simulink model "W07_0_offline"  (R2024b)
settings: Solver=ode4  StartTime=0.0  StopTime=600  FixedStep=Ts_ctrl  RelTol=1e-3
values from neighbouring files (symbols this model uses):
  animate = 0    [W05_compare.m]    (also in W05_crab_demo.m; W05_lookahead_demo.m; W05_setup.m = 1; W07_setup.m = 1)
  beta_c = deg2rad(current_direction)    [W05_compare.m]    (also in W05_crab_demo.m; W05_setup.m; W07_setup.m)
  current_speed = CASES{i,3}    [W05_compare.m]    (also in W05_crab_demo.m = CUR(i); W05_setup.m = 0; W07_setup.m = 0)
  d_mode = 1    [W07_setup.m]
  Delta = DELTAS(i)    [W05_lookahead_demo.m]    (also in W05_setup.m = 10; W07_setup.m = 10)
  F_max = 500    [W05_setup.m]    (also in W07_setup.m)
  guidance_mode = CASES{i,2}    [W05_compare.m]    (also in W05_setup.m = 2; W07_setup.m = 2)
  half_beam = 1.027135    [W05_setup.m]    (also in W07_setup.m)
  Izz = 653    [W05_setup.m]    (also in W07_setup.m; build_w05_models.m = p(2))
  k_prop = 1000 * 0.004422 * 0.2^4    (= 0.0070752)    [W05_setup.m]    (also in W07_setup.m)
  Kd_psi = 200    [W05_setup.m]    (also in W07_setup.m)
  Ki_u = 100    [W05_setup.m]    (also in W07_setup.m)
  Kp_psi = 400    [W05_setup.m]    (also in W07_setup.m)
  Kp_u = 300    [W05_setup.m]    (also in W07_setup.m)
  m_usv = 211    [W05_setup.m]    (also in W07_setup.m)
  n_max = sqrt(F_max / k_prop)    [W05_setup.m]    (also in W07_setup.m)
  Nr = 800    [W05_setup.m]    (also in W07_setup.m)
  Nrr = 800    [W05_setup.m]    (also in W07_setup.m; build_w05_models.m = p(8))
  R_LOS = 5    [W05_lookahead_demo.m]    (also in W05_setup.m; W07_setup.m)
  sw_mode = 1    [W05_lookahead_demo.m]    (also in W05_setup.m; W07_setup.m)
  tau_n = 0.30    (= 0.3)    [W05_setup.m]    (also in W07_setup.m)
  Ts_ctrl = 0.05    [W05_setup.m]    (also in W07_setup.m)
  u_ref = 1.5    [W05_setup.m]    (also in W07_setup.m)
  wp_east = [  20   20  100  100   20 ]    [W05_setup.m]    (also in W07_setup.m)
  wp_north = [ -20   60   60  -20  -20 ]    [W05_setup.m]    (also in W07_setup.m)
  x0 = [0.1; 0; 0; 0; 0; psi_init]    [W05_setup.m]    (also in W05_vrx_run.m = x0old;   x0(6) = psi0;   assignin('base','x0', x0); W07_setup.m)
  Xu = 100    [W05_setup.m]    (also in W07_setup.m; build_w05_models.m = p(3))
  Xuu = 150    [W05_setup.m]    (also in W07_setup.m; build_w05_models.m = p(4))
  Yv = 100    [W05_setup.m]    (also in W07_setup.m; build_w05_models.m = p(5))
  Yvv = 100    [W05_setup.m]    (also in W07_setup.m; build_w05_models.m = p(6);'                newline  'Nr=p(7))
libraries: slpidlib x1, simulink x1
settings Model: Creator=admin  LastModifiedBy=admin

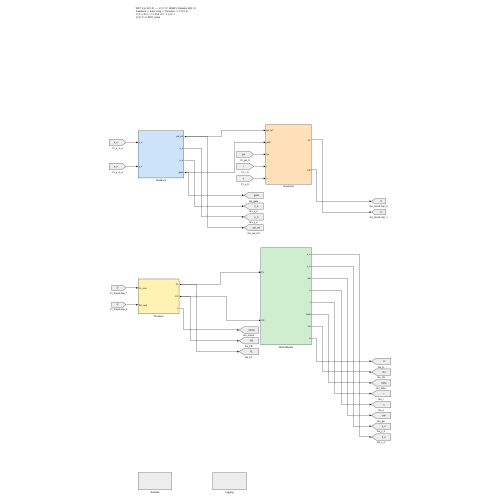
[thumbnail: Simulink's stored preview of the top-level diagram]
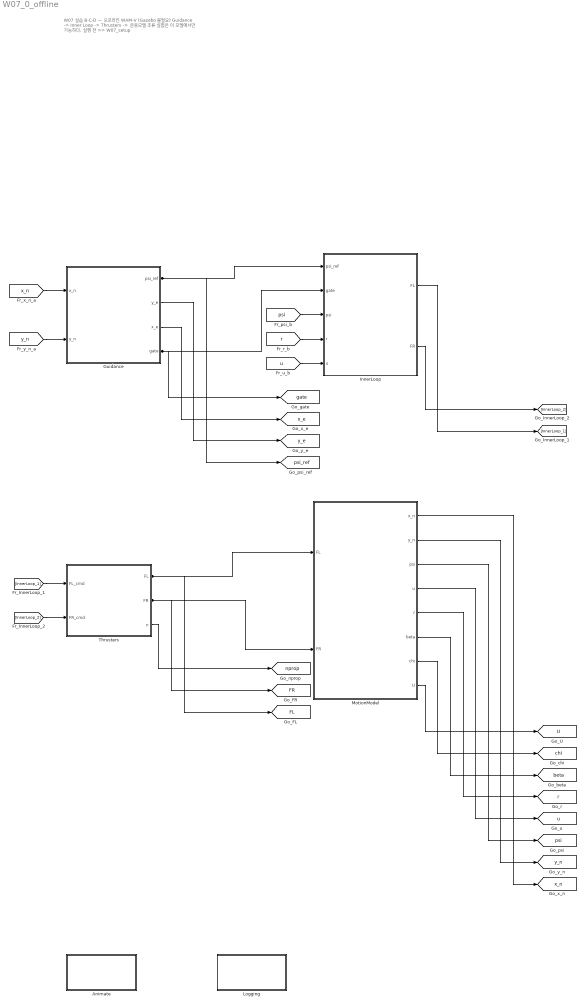
== system W07_0_offline ==
  note: W07 실습 B·C·D  —  오프라인 WAM-V (Gazebo 불필요)
      | Guidance -> Inner Loop -> Thrusters -> 운동모델
      | 조류 실험은 이 모델에서만 가능하다.
      | 실행 전 >> W07_setup
  Animate : Subsystem
  Guidance : Subsystem
  InnerLoop : Subsystem
  Logging : Subsystem
  MotionModel : Subsystem
  Thrusters : Subsystem
  tag scope: FL=global, FR=global, U=global, beta=global, chi=global, gate=global, nprop=global, psi=global, psi_ref=global, r=global, u=global, x_e=global, x_n=global, y_e=global, y_n=global
  wires:
  MotionModel/8(U) -> [U]
  MotionModel/7(chi) -> [chi]
  MotionModel/6(beta) -> [beta]
  MotionModel/5(r) -> [r]
  MotionModel/4(u) -> [u]
  MotionModel/3(psi) -> [psi]
  MotionModel/2(y_n) -> [y_n]
  MotionModel/1(x_n) -> [x_n]
  InnerLoop/2(FR) -> [InnerLoop_2]
  InnerLoop/1(FL) -> [InnerLoop_1]
  Thrusters/3(n) -> [nprop]
  Thrusters/2(FR) -> MotionModel/2(FR), [FR]
  Thrusters/1(FL) -> MotionModel/1(FL), [FL]
  [u] -> InnerLoop/5(u)
  [r] -> InnerLoop/4(r)
  [psi] -> InnerLoop/3(psi)
  Guidance/4(gate) -> InnerLoop/2(gate), [gate]
  Guidance/3(x_e) -> [x_e]
  Guidance/2(y_e) -> [y_e]
  Guidance/1(psi_ref) -> InnerLoop/1(psi_ref), [psi_ref]
  [y_n] -> Guidance/2(y_n)
  [x_n] -> Guidance/1(x_n)
  [InnerLoop_2] -> Thrusters/2(FR_cmd)
  [InnerLoop_1] -> Thrusters/1(FL_cmd)

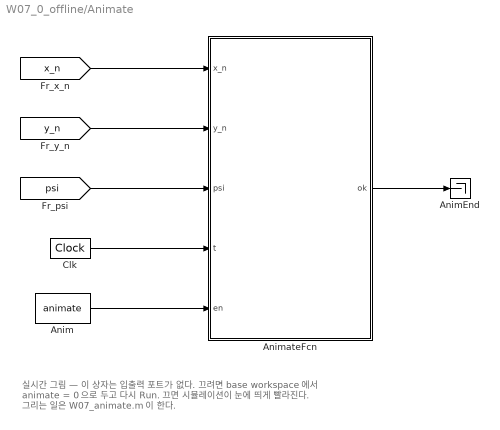
== system W07_0_offline/Animate ==
  note: 실시간 그림 — 이 상자는 입출력 포트가 없다.
      | 끄려면 base workspace 에서  animate = 0  으로 두고 다시 Run.
      | 끄면 시뮬레이션이 눈에 띄게 빨라진다.
      | 그리는 일은 W07_animate.m 이 한다.
  Anim : Constant  Value=animate
  AnimEnd : Terminator
  AnimateFcn : MATLAB Function  TreatAsAtomicUnit=on
  Clk : DigitalClock  SampleTime=Ts_ctrl
  wires:
  [x_n] -> AnimateFcn/1(x_n)
  [y_n] -> AnimateFcn/2(y_n)
  [psi] -> AnimateFcn/3(psi)
  Clk/1 -> AnimateFcn/4(t)
  Anim/1 -> AnimateFcn/5(en)
  AnimateFcn/1(ok) -> AnimEnd/1

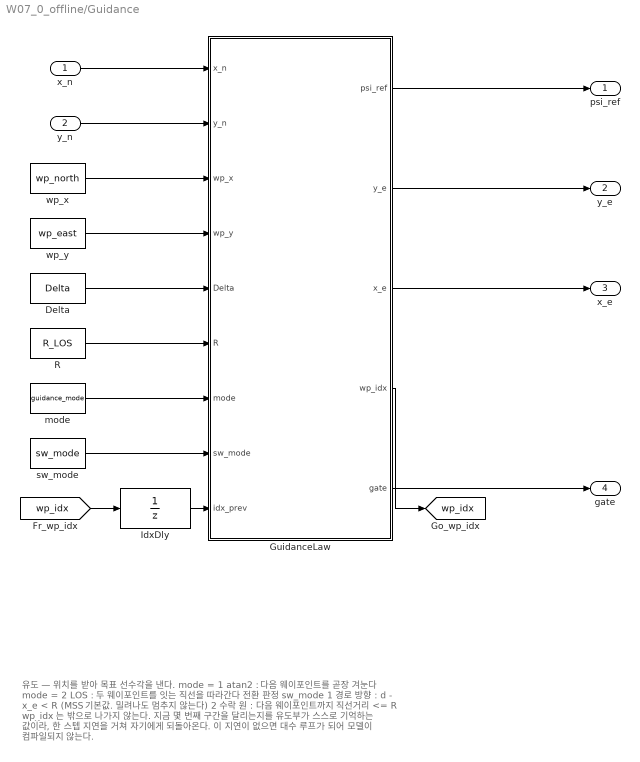
== system W07_0_offline/Guidance ==
  note: 유도 — 위치를 받아 목표 선수각을 낸다.
      |   mode = 1  atan2 : 다음 웨이포인트를 곧장 겨눈다
      |   mode = 2  LOS   : 두 웨이포인트를 잇는 직선을 따라간다
      |
      | 전환 판정 sw_mode
      |   1  경로 방향 : d - x_e < R   (MSS 기본값. 밀려나도 멈추지 않는다)
      |   2  수락 원   : 다음 웨이포인트까지 직선거리 <= R
      |
      | wp_idx 는 밖으로 나가지 않는다. 지금 몇 번째 구간을 달리는지를
      | 유도부가 스스로 기억하는 값이라, 한 스텝 지연을 거쳐 자기에게 되돌아온다.
      | 이 지연이 없으면 대수 루프가 되어 모델이 컴파일되지 않는다.
  x_n : Inport
  y_n : Inport  Port=2
  Delta : Constant  Value=Delta
  GuidanceLaw : MATLAB Function  TreatAsAtomicUnit=on
  IdxDly : UnitDelay  InitialCondition=1  SampleTime=Ts_ctrl  HasFrameUpgradeWarning=on
  R : Constant  Value=R_LOS
  mode : Constant  Value=guidance_mode
  sw_mode : Constant  Value=sw_mode
  wp_x : Constant  Value=wp_north
  wp_y : Constant  Value=wp_east
  psi_ref : Outport
  y_e : Outport  Port=2
  x_e : Outport  Port=3
  gate : Outport  Port=4
  tag scope: wp_idx=global
  wires:
  x_n/1 -> GuidanceLaw/1(x_n)
  y_n/1 -> GuidanceLaw/2(y_n)
  wp_x/1 -> GuidanceLaw/3(wp_x)
  wp_y/1 -> GuidanceLaw/4(wp_y)
  Delta/1 -> GuidanceLaw/5(Delta)
  R/1 -> GuidanceLaw/6(R)
  mode/1 -> GuidanceLaw/7(mode)
  sw_mode/1 -> GuidanceLaw/8(sw_mode)
  [wp_idx] -> IdxDly/1
  IdxDly/1 -> GuidanceLaw/9(idx_prev)
  GuidanceLaw/1(psi_ref) -> psi_ref/1
  GuidanceLaw/2(y_e) -> y_e/1
  GuidanceLaw/3(x_e) -> x_e/1
  GuidanceLaw/5(gate) -> gate/1
  GuidanceLaw/4(wp_idx) -> [wp_idx]

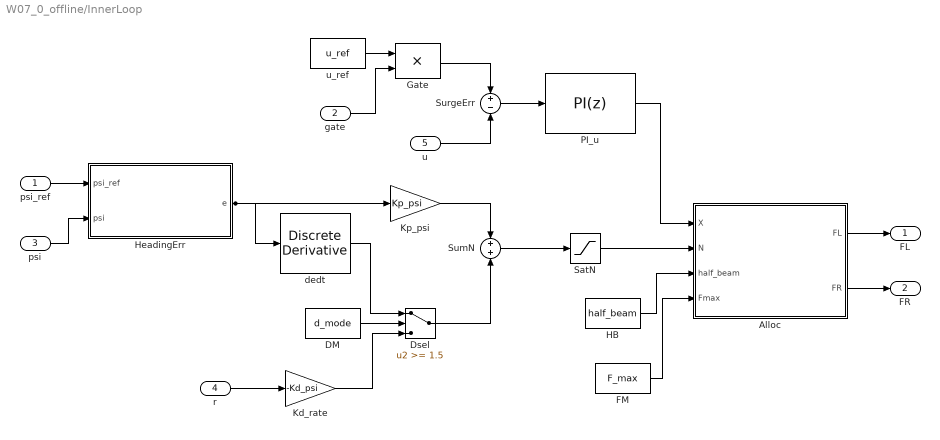
== system W07_0_offline/InnerLoop ==
  psi_ref : Inport
  gate : Inport  Port=2
  psi : Inport  Port=3
  r : Inport  Port=4
  u : Inport  Port=5
  Alloc : MATLAB Function  TreatAsAtomicUnit=on
  DM : Constant  Value=d_mode
  Dsel : Switch  Threshold=1.5  SaturateOnIntegerOverflow=off  InputSameDT=off
  FM : Constant  Value=F_max
  Gate : Product
  HB : Constant  Value=half_beam
  HeadingErr : MATLAB Function  TreatAsAtomicUnit=on
  Kd_rate : Gain  Gain=-Kd_psi
  Kp_psi : Gain  Gain=Kp_psi
  PI_u : slpidlib/PID Controller  Controller=PI  Form=Parallel  TimeDomain=Discrete-time  UseExternalTs=off  SampleTime=Ts_ctrl  IntegratorMethod=Forward Euler  FilterMethod=Forward Euler  ControllerParametersSource=internal  P=Kp_u  I=Ki_u  UseKiTs=off  D=0  UseExternalDerivativeSource=off  N=100  UseFilter=on  TunerSelectOption=Transfer Function Based (PID Tuner App)  InitialConditionSource=internal  InitialConditionForIntegrator=0  InitialConditionForFilter=0  DifferentiatorICPrevScaledInput=0  ExternalReset=none  TrackingMode=off  Kt=1  LimitOutput=on  SatLimitsSource=internal  UpperSaturationLimit=2*F_max  LowerSaturationLimit=-2*F_max  LinearizeAsGain=on  AntiWindupMode=clamping  Kb=1  LimitIntegrator=off  UpperIntegratorSaturationLimit=inf  LowerIntegratorSaturationLimit=-inf  POutMin=[]  POutMax=[]  IOutMin=[]  IOutMax=[]  DOutMin=[]  DOutMax=[]  NOutMin=[]  NOutMax=[]  SumOutMin=[]  SumOutMax=[]  SaturationOutMin=[]  SaturationOutMax=[]  PParamMin=[]  PParamMax=[]  IParamMin=[]  IParamMax=[]  DParamMin=[]  DParamMax=[]  NParamMin=[]  NParamMax=[]  KbParamMin=[]  KbParamMax=[]  KtParamMin=[]  KtParamMax=[]  KbOutMin=[]  KbOutMax=[]  KtOutMin=[]  KtOutMax=[]  IntegratorOutMin=[]  IntegratorOutMax=[]  FilterOutMin=[]  FilterOutMax=[]  SumI1OutMin=[]  SumI1OutMax=[]  SumI2OutMin=[]  SumI2OutMax=[]  SumI3OutMin=[]  SumI3OutMax=[]  SumI4OutMin=[]  SumI4OutMax=[]  SumDOutMin=[]  SumDOutMax=[]  DifferentiatorOutMin=[]  DifferentiatorOutMax=[]  FilterDiffOutCoefMin=[]  FilterDiffOutCoefMax=[]  ReciprocalOutMin=[]  ReciprocalOutMax=[]  SumDenOutMin=[]  SumDenOutMax=[]  SumNumOutMin=[]  SumNumOutMax=[]  DivideOutMin=[]  DivideOutMax=[]  UdiffTsProdOutMin=[]  UdiffTsProdOutMax=[]  NTsProdOutMin=[]  NTsProdOutMax=[]  UintegralTsProdOutMin=[]  UintegralTsProdOutMax=[]  UngainTsProdOutMin=[]  UngainTsProdOutMax=[]  ClampingZeroOutDataTypeStr=Inherit: Inherit via back propagation  ClampingZeroOutMin=[]  ClampingZeroOutMax=[]  FilterDenConstantOutDataTypeStr=Inherit: Inherit via back propagation  FilterDenConstantOutMin=[]  FilterDenConstantOutMax=[]  PCopyOutDataTypeStr=Inherit: Inherit via back propagation  PCopyOutMin=[]  PCopyOutMax=[]  NCopyOutDataTypeStr=Inherit: Inherit via back propagation  NCopyOutMin=[]  NCopyOutMax=[]  IntegratorContinuousStateAttributes=''  IntegratorStateMustResolveToSignalObject=off  IntegratorRTWStateStorageClass=Auto  FilterContinuousStateAttributes=''  FilterStateMustResolveToSignalObject=off  FilterRTWStateStorageClass=Auto  ParallelPVariant=InternalParameters  IdealPVariant=Disabled  IVariant=InternalParameters  DVariant=Disabled  IntegratorVariant=Discrete  SatVariant=Enabled  AWVariant=DiscClampingParallel  PCopyVariant=Disabled  TRVariant=Disabled  FdbkBlocksVariant=Forward  IdealPFdbkVariant=Disabled  SatFdbkVariant=Disabled  DerivativeFilterVariant=Disabled  NVariant=Disabled  NCopyVariant=Disabled_SignalSpec  FilterICVariant=Disabled  IntegratorICVariant=InternalICs  ExternalResetVariant=Disabled  TRSumVariant=Passthrough  SumFdbkVariant=Disabled  SumVariant=Sum_PI  TsampFilterVariant=InternalTs  TsampNgainVariant=Passthrough  TsampIntegralVariant=Disabled_SignalSpec  ExternalSaturationOutDataTypeStr=Inherit: Same as second input  DerivativeSourceVariant=Disabled  PreIntVariant=InternalPreInt
  SatN : Saturate  UpperLimit=2*F_max*half_beam  LowerLimit=-2*F_max*half_beam
  SumN : Sum
  SurgeErr : Sum  Inputs=+-
  dedt : simulink/Discrete/Discrete Derivative  gainval=Kd_psi  ICPrevScaledInput=0.0  OutMin=[]  OutMax=[]  OutDataType=fixdt(1, 16)  OutScaling=2^-10  DoSatur=off
  u_ref : Constant  Value=u_ref
  FL : Outport
  FR : Outport  Port=2
  wires:
  gate/1 -> Gate/2
  psi_ref/1 -> HeadingErr/1(psi_ref)
  dedt/1 -> Dsel/1
  r/1 -> Kd_rate/1
  psi/1 -> HeadingErr/2(psi)
  HeadingErr/1(e) -> dedt/1, Kp_psi/1
  u_ref/1 -> Gate/1
  Alloc/1(FL) -> FL/1
  DM/1 -> Dsel/2
  Kd_rate/1 -> Dsel/3
  Gate/1 -> SurgeErr/1
  u/1 -> SurgeErr/2
  Kp_psi/1 -> SumN/1
  Dsel/1 -> SumN/2
  SurgeErr/1 -> PI_u/1
  SumN/1 -> SatN/1
  PI_u/1 -> Alloc/1(X)
  SatN/1 -> Alloc/2(N)
  HB/1 -> Alloc/3(half_beam)
  Alloc/2(FR) -> FR/1
  FM/1 -> Alloc/4(Fmax)

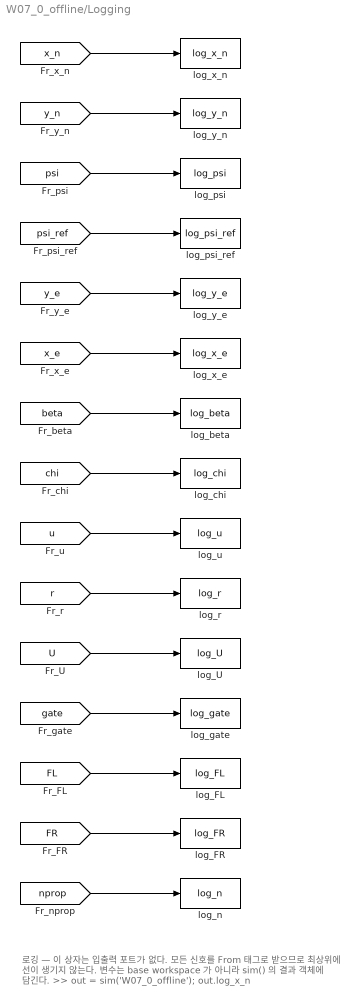
== system W07_0_offline/Logging ==
  note: 로깅 — 이 상자는 입출력 포트가 없다.
      | 모든 신호를 From 태그로 받으므로 최상위에 선이 생기지 않는다.
      | 변수는 base workspace 가 아니라 sim() 의 결과 객체에 담긴다.
      |   >> out = sim('W07_0_offline');  out.log_x_n
  log_FL : ToWorkspace  VariableName=log_FL  SaveFormat=Timeseries  SampleTime=Ts_ctrl
  log_FR : ToWorkspace  VariableName=log_FR  SaveFormat=Timeseries  SampleTime=Ts_ctrl
  log_U : ToWorkspace  VariableName=log_U  SaveFormat=Timeseries  SampleTime=Ts_ctrl
  log_beta : ToWorkspace  VariableName=log_beta  SaveFormat=Timeseries  SampleTime=Ts_ctrl
  log_chi : ToWorkspace  VariableName=log_chi  SaveFormat=Timeseries  SampleTime=Ts_ctrl
  log_gate : ToWorkspace  VariableName=log_gate  SaveFormat=Timeseries  SampleTime=Ts_ctrl
  log_n : ToWorkspace  VariableName=log_n  SaveFormat=Timeseries  SampleTime=Ts_ctrl
  log_psi : ToWorkspace  VariableName=log_psi  SaveFormat=Timeseries  SampleTime=Ts_ctrl
  log_psi_ref : ToWorkspace  VariableName=log_psi_ref  SaveFormat=Timeseries  SampleTime=Ts_ctrl
  log_r : ToWorkspace  VariableName=log_r  SaveFormat=Timeseries  SampleTime=Ts_ctrl
  log_u : ToWorkspace  VariableName=log_u  SaveFormat=Timeseries  SampleTime=Ts_ctrl
  log_x_e : ToWorkspace  VariableName=log_x_e  SaveFormat=Timeseries  SampleTime=Ts_ctrl
  log_x_n : ToWorkspace  VariableName=log_x_n  SaveFormat=Timeseries  SampleTime=Ts_ctrl
  log_y_e : ToWorkspace  VariableName=log_y_e  SaveFormat=Timeseries  SampleTime=Ts_ctrl
  log_y_n : ToWorkspace  VariableName=log_y_n  SaveFormat=Timeseries  SampleTime=Ts_ctrl
  wires:
  [x_n] -> log_x_n/1
  [y_n] -> log_y_n/1
  [psi] -> log_psi/1
  [psi_ref] -> log_psi_ref/1
  [y_e] -> log_y_e/1
  [x_e] -> log_x_e/1
  [beta] -> log_beta/1
  [chi] -> log_chi/1
  [u] -> log_u/1
  [r] -> log_r/1
  [U] -> log_U/1
  [gate] -> log_gate/1
  [FL] -> log_FL/1
  [FR] -> log_FR/1
  [nprop] -> log_n/1

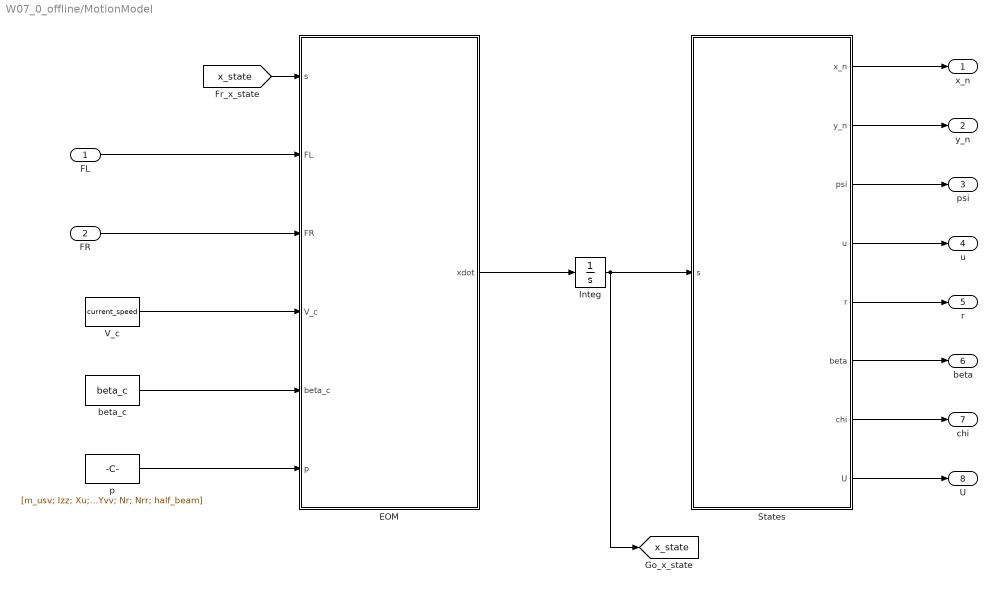
== system W07_0_offline/MotionModel ==
  FL : Inport
  FR : Inport  Port=2
  EOM : MATLAB Function  TreatAsAtomicUnit=on
  Integ : Integrator  InitialCondition=x0
  States : MATLAB Function  TreatAsAtomicUnit=on
  V_c : Constant  Value=current_speed
  beta_c : Constant  Value=beta_c
  p : Constant  Value=[m_usv; Izz; Xu; Xuu; Yv; Yvv; Nr; Nrr; half_beam]
  x_n : Outport
  y_n : Outport  Port=2
  psi : Outport  Port=3
  u : Outport  Port=4
  r : Outport  Port=5
  beta : Outport  Port=6
  chi : Outport  Port=7
  U : Outport  Port=8
  tag scope: x_state=global
  wires:
  FL/1 -> EOM/2(FL)
  FR/1 -> EOM/3(FR)
  V_c/1 -> EOM/4(V_c)
  beta_c/1 -> EOM/5(beta_c)
  p/1 -> EOM/6(p)
  EOM/1(xdot) -> Integ/1
  Integ/1 -> States/1(s), [x_state]
  [x_state] -> EOM/1(s)
  States/1(x_n) -> x_n/1
  States/2(y_n) -> y_n/1
  States/3(psi) -> psi/1
  States/4(u) -> u/1
  States/5(r) -> r/1
  States/6(beta) -> beta/1
  States/7(chi) -> chi/1
  States/8(U) -> U/1

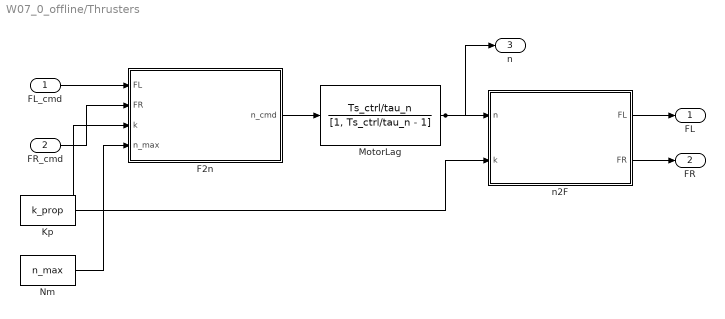
== system W07_0_offline/Thrusters ==
  FL_cmd : Inport
  FR_cmd : Inport  Port=2
  F2n : MATLAB Function  TreatAsAtomicUnit=on
  Kp : Constant  Value=k_prop
  MotorLag : DiscreteTransferFcn  Numerator=Ts_ctrl/tau_n  Denominator=[1, Ts_ctrl/tau_n - 1]  SampleTime=Ts_ctrl
  Nm : Constant  Value=n_max
  n2F : MATLAB Function  TreatAsAtomicUnit=on
  FL : Outport
  FR : Outport  Port=2
  n : Outport  Port=3
  wires:
  n2F/1(FL) -> FL/1
  FR_cmd/1 -> F2n/2(FR)
  FL_cmd/1 -> F2n/1(FL)
  Kp/1 -> n2F/2(k), F2n/3(k)
  Nm/1 -> F2n/4(n_max)
  F2n/1(n_cmd) -> MotorLag/1
  MotorLag/1 -> n/1, n2F/1(n)
  n2F/2(FR) -> FR/1

== matlab function W07_0_offline/Animate/AnimateFcn ==
  data: x_n input; ok output; y_n input; psi input; t input; en input
function ok = AnimateFcn(x_n, y_n, psi, t, en)
%#codegen
% Live plot while the model runs. A MATLAB Function block cannot
% plot, so the drawing function is declared extrinsic: Simulink
% calls plain MATLAB instead of generating code for it.
coder.extrinsic('W07_animate');
ok = 1;
if en > 0.5
    W07_animate(x_n, y_n, psi, t);
end

== matlab function W07_0_offline/InnerLoop/HeadingErr ==
  data: psi_ref input; e output; psi input
function e = HeadingErr(psi_ref, psi)
%#codegen
% Shortest signed angle (ssa). Without it a command of 179 deg
% against a heading of -179 deg reads as a 358 deg error and
% the boat turns the long way round.
d = psi_ref - psi;
e = atan2(sin(d), cos(d));

== matlab function W07_0_offline/Guidance/GuidanceLaw ==
  data: x_n input; psi_ref output; y_n input; wp_x input; wp_y input; Delta input; R input; mode input; sw_mode input; idx_prev input; y_e output; x_e output; wp_idx output; gate output
function [psi_ref, y_e, x_e, wp_idx, gate] = GuidanceLaw(x_n, y_n, wp_x, wp_y, Delta, R, mode, sw_mode, idx_prev)
%#codegen
% Waypoint guidance. Two laws in one block. Both return a HEADING command,
% following the MSS demo demoOtterUSVHeadingControl.slx and GNC/LOSchi.m.
%   mode 1 = atan2 : aim straight at the next waypoint (point chasing)
%   mode 2 = LOS   : follow the straight line between two waypoints
% Switching criterion (sw_mode):
%   1 = along-track : d - x_e < R      (MSS / Fossen default, cannot hang)
%   2 = circle      : distance to the next waypoint <= R

n = numel(wp_x);
k = min(max(idx_prev, 1), n-1);        % index of the active leg

xk  = wp_x(k);    yk  = wp_y(k);       % leg start
xk1 = wp_x(k+1);  yk1 = wp_y(k+1);     % leg end = next waypoint

% path-tangential angle of the active leg, measured from North
pi_p = atan2(yk1 - yk, xk1 - xk);

% Both errors come out of ONE rotation of (p - p_k) into the path frame.
% x_e = how far ALONG the leg,  y_e = how far TO THE SIDE of it.
% Computed the same way for BOTH guidance laws so that the two can be
% compared with the same yardstick.
x_e =  (x_n - xk)*cos(pi_p) + (y_n - yk)*sin(pi_p);
y_e = -(x_n - xk)*sin(pi_p) + (y_n - yk)*cos(pi_p);

if mode == 1
    psi_ref = atan2(yk1 - y_n, xk1 - x_n);
else
    psi_ref = pi_p - atan(y_e / Delta);
end

% --- waypoint switching ---------------------------------------------
% d is the leg length, so d - x_e is the along-track distance REMAINING.
% The circle test is always the stricter of the two, because
%     distance = sqrt((d - x_e)^2 + y_e^2) >= d - x_e
% A boat blown wide of a waypoint never enters that circle, and a mission
% that waits for it waits for ever. The along-track test cannot hang.
d = sqrt((xk1 - xk)^2 + (yk1 - yk)^2);
if sw_mode == 1
    reached = (d - x_e) < R;
else
    reached = sqrt((xk1 - x_n)^2 + (yk1 - y_n)^2) <= R;
end

% wp_idx = n means "mission finished" and it LATCHES: once the last leg is
% done, the boat stays stopped even if the current pushes it back behind the
% finish line (then reached would turn false again).
if idx_prev >= n
    wp_idx = n;                         % already finished - stay finished
elseif reached && (k < n-1)
    wp_idx = k + 1;
elseif reached && (k == n-1)
    wp_idx = n;                         % last leg done
else
    wp_idx = k;
end

% gate = 0 brings the boat to a stop. Without it the boat would follow the
% last leg forever.
gate = double(wp_idx < n);

== matlab function W07_0_offline/InnerLoop/Alloc ==
  data: X input; FL output; N input; half_beam input; Fmax input; FR output
function [FL, FR] = Alloc(X, N, half_beam, Fmax)
%#codegen
% Differential thrust allocation for two aft thrusters.
%   X = FL + FR              surge force [N]
%   N = (FL - FR)*half_beam  yaw moment  [N*m]
FL = X/2 + N/(2*half_beam);
FR = X/2 - N/(2*half_beam);
if FL >  Fmax, FL =  Fmax; end
if FL < -Fmax, FL = -Fmax; end
if FR >  Fmax, FR =  Fmax; end
if FR < -Fmax, FR = -Fmax; end

== matlab function W07_0_offline/Thrusters/F2n ==
  data: FL input; n_cmd output; FR input; k input; n_max input
function n_cmd = F2n(FL, FR, k, n_max)
%#codegen
% Inverse propeller law: turn a demanded thrust into a shaft speed.
%   F = k*n*|n|   ->   n = sign(F)*sqrt(|F|/k)
% Saturation happens on SPEED, not on force. That is what a real
% motor limits.
F = [FL; FR];
n_cmd = zeros(2,1);
for i = 1:2
    ni = sign(F(i)) * sqrt(abs(F(i))/k);
    if ni >  n_max, ni =  n_max; end
    if ni < -n_max, ni = -n_max; end
    n_cmd(i) = ni;
end

== matlab function W07_0_offline/Thrusters/n2F ==
  data: n input; FL output; k input; FR output
function [FL, FR] = n2F(n, k)
%#codegen
% Forward propeller law. Note the |n| : thrust is quadratic in
% shaft speed, so a rate limit on n is NOT a rate limit on F.
FL = k * n(1) * abs(n(1));
FR = k * n(2) * abs(n(2));

== matlab function W07_0_offline/MotionModel/EOM ==
  data: s input; xdot output; FL input; FR input; V_c input; beta_c input; p input
function xdot = EOM(s, FL, FR, V_c, beta_c, p)
%#codegen
% 3-DOF WAM-V equations of motion, NED.
% Coefficients come straight from the Gazebo VRX plugins:
%   drag       : SimpleHydrodynamics  (Xu Xuu Yv Yvv Nr Nrr)
%   mass       : wamv_base.urdf.xacro (180 kg hull + engines)
%   added mass : zero in VRX (xDotU = yDotV = nDotR = 0)
% Ocean current exists only here. Gazebo has no current plugin.
%   s = [u v r N E psi]'
%   p = [m Izz Xu Xuu Yv Yvv Nr Nrr half_beam]'

u = s(1); v = s(2); r = s(3); psi = s(6);
m=p(1); Izz=p(2); Xu=p(3); Xuu=p(4); Yv=p(5); Yvv=p(6);
Nr=p(7); Nrr=p(8); b_half=p(9);

% current in the body frame -> velocity relative to the water
u_c = V_c*cos(beta_c - psi);
v_c = V_c*sin(beta_c - psi);
u_r = u - u_c;
v_r = v - v_c;

% differential thrust -> surge force and yaw moment
X = FL + FR;
N = (FL - FR)*b_half;

% drag acts on the velocity relative to the water
Dx = (Xu + Xuu*abs(u_r))*u_r;
Dy = (Yv + Yvv*abs(v_r))*v_r;
Dn = (Nr + Nrr*abs(r))*r;

du = (X - Dx)/m + v*r;      % rigid-body Coriolis
dv = (  - Dy)/m - u*r;
dr = (N - Dn)/Izz;

xdot = [du; dv; dr;
        u*cos(psi) - v*sin(psi);   % kinematics use absolute velocity
        u*sin(psi) + v*cos(psi);
        r];

== matlab function W07_0_offline/MotionModel/States ==
  data: s input; x_n output; y_n output; psi output; u output; r output; beta output; chi output; U output
function [x_n, y_n, psi, u, r, beta, chi, U] = States(s)
%#codegen
% Pick the navigation quantities out of the state vector.
% In the VRX model this job is done by the Nav block,
% which also has to convert ENU to NED.
u = s(1); v = s(2); r = s(3);
x_n = s(4); y_n = s(5); psi = s(6);
U    = sqrt(u*u + v*v);      % speed over ground
beta = atan2(v, u);          % crab angle
c    = psi + beta;           % course angle
chi  = atan2(sin(c), cos(c));
